simulink model "Q3"  (R2021a)
settings: Solver=VariableStepAuto  StartTime=0.0  StopTime=10.0  RelTol=1e-3
settings Model: Creator=WH  LastModifiedBy=WH

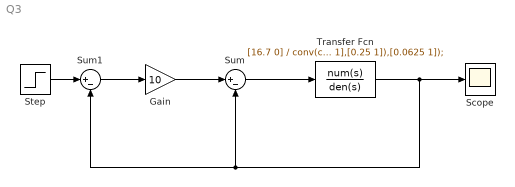
== system Q3 ==
  Gain : Gain  Gain=10
  Scope : Scope
  Step : Step  SampleTime=0
  Sum : Sum  Inputs=|+-
  Sum1 : Sum  Inputs=|+-
  Transfer Fcn : TransferFcn  Numerator=[16.7 0]  Denominator=conv(conv([0.85 1],[0.25 1]),[0.0625 1]);
  wires:
  Sum/1 -> Transfer Fcn/1
  Gain/1 -> Sum/1
  Step/1 -> Sum1/1
  Sum1/1 -> Gain/1
  Transfer Fcn/1 -> Sum1/2, Sum/2, Scope/1
